simulink model "ModelTestVersion"  (Simulink 9.2)
settings: Solver=FixedStepAuto  StartTime=0.0  StopTime=30  FixedStep=0.01  RelTol=1e-3
values from neighbouring files (symbols this model uses):
  I = 1    [Initialization.m]
  Ke = 6.67*10e-4    (= 0.00667)    [Initialization.m]
  Kec = 8.33*10e-5    (= 0.000833)    [Initialization.m]
  Ki = 0.01    [Initialization.m]
  Kp = 0.015    [Initialization.m]
  P = 5    [Initialization.m]
libraries: simulink x2, fuzblock x1
settings Model: Creator=zelex  LastModifiedBy=zelex
settings DataIOCC: LimitDataPoints=off  SaveFormat=Dataset  SignalLoggingSaveFormat=Dataset
settings OptimizationCC: LifeSpan=auto
settings DebuggingCC: UnderspecifiedInitializationDetection=Simplified  MergeDetectMultiDrivingBlocksExec=error  FcnCallInpInsideContextMsg=error  StateNameClashWarn=none  SFUnexpectedBacktrackingDiag=error  SFNoUnconditionalDefaultTransitionDiag=error
settings HardwareCC: ProdBitPerPointer=64  ProdBitPerSizeT=64  ProdBitPerPtrDiffT=64  ProdLargestAtomicFloat=Float  ProdIntDivRoundTo=Zero  ProdEndianess=LittleEndian  ProdWordSize=64  ProdHWDeviceType=Intel->x86-64 (Windows64)
settings ModelReferenceCC: PropagateSignalLabelsOutOfModel=on
settings SFSimCC: SimUseLocalCustomCode=on
settings RTWCC: RTWUseLocalCustomCode=on
settings GRTTargetCC: GeneratePreprocessorConditionals=Use local settings  CombineOutputUpdateFcns=on  GRTInterface=off

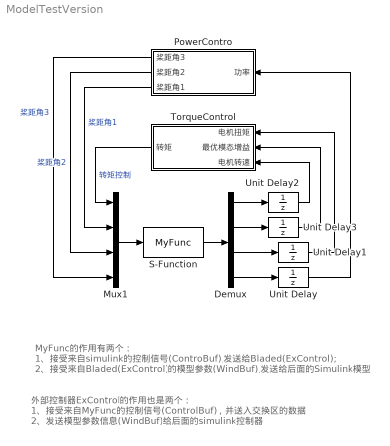
== system ModelTestVersion ==
  note: 外部控制器ExControl的作用也是两个：
      | 1、接受来自MyFunc的控制信号(ControlBuf)，并送入交换区的数据
      | 2、发送模型参数信息(WindBuf)给后面的simulink控制器
  note: MyFunc的作用有两个：
      | 1、接受来自simulink的控制信号(ControBuf),发送给Bladed(ExControl);
      | 2、接受来自Bladed(ExControl)的模型参数(WindBuf),发送给后面的Simulink模型
  Demux : Demux
  Mux1 : Mux
  PowerContro : Subsystem
  S-Function : S-Function  FunctionName=MyFunc  SFunctionDeploymentMode=off  EnableBusSupport=off
  TorqueControl : Subsystem
  Unit Delay : UnitDelay  SampleTime=0.01
  Unit Delay1 : UnitDelay  SampleTime=0.01
  Unit Delay2 : UnitDelay  SampleTime=0.01
  Unit Delay3 : UnitDelay  InitialCondition=22.82  SampleTime=0.01
  wires:
  Mux1/1 -> S-Function/1
  TorqueControl/1(转矩) -> Mux1/1  "转矩控制"
  PowerContro/3(桨距角1) -> Mux1/2  "桨距角1"
  PowerContro/2(桨距角2) -> Mux1/3  "桨距角2"
  PowerContro/1(桨距角3) -> Mux1/4  "桨距角3"
  S-Function/1 -> Demux/1
  Demux/1 -> Unit Delay2/1
  Demux/2 -> Unit Delay3/1
  Demux/3 -> Unit Delay1/1
  Demux/4 -> Unit Delay/1
  Unit Delay2/1 -> TorqueControl/3(电机转速)
  Unit Delay3/1 -> TorqueControl/2(最优模态增益)
  Unit Delay1/1 -> TorqueControl/1(电机扭矩)
  Unit Delay/1 -> PowerContro/1(功率)

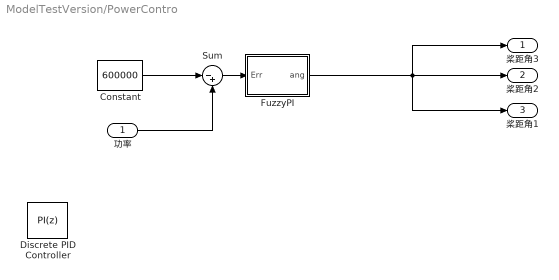
== system ModelTestVersion/PowerContro ==
  功率 : Inport
  Constant : Constant  Value=600000
  Discrete PID Controller : simulink/Continuous/PID Controller  Controller=PI  Form=Ideal  TimeDomain=Discrete-time  SampleTime=-1  IntegratorMethod=Forward Euler  FilterMethod=Forward Euler  ControllerParametersSource=internal  P=0.5  I=10  D=0  UseFilter=on  N=100  TunerSelectOption=Transfer Function Based (PID Tuner App)  InitialConditionSource=internal  InitialConditionForIntegrator=0  InitialConditionForFilter=0  DifferentiatorICPrevScaledInput=0  ExternalReset=none  TrackingMode=off  Kt=1  LimitOutput=off  UpperSaturationLimit=inf  LowerSaturationLimit=-inf  LinearizeAsGain=off  AntiWindupMode=none  Kb=1  POutMin=[]  POutMax=[]  IOutMin=[]  IOutMax=[]  DOutMin=[]  DOutMax=[]  NOutMin=[]  NOutMax=[]  SumOutMin=[]  SumOutMax=[]  SaturationOutMin=[]  SaturationOutMax=[]  PParamMin=[]  PParamMax=[]  IParamMin=[]  IParamMax=[]  DParamMin=[]  DParamMax=[]  NParamMin=[]  NParamMax=[]  KbParamMin=[]  KbParamMax=[]  KtParamMin=[]  KtParamMax=[]  KbOutMin=[]  KbOutMax=[]  KtOutMin=[]  KtOutMax=[]  IntegratorOutMin=[]  IntegratorOutMax=[]  FilterOutMin=[]  FilterOutMax=[]  SumI1OutMin=[]  SumI1OutMax=[]  SumI2OutMin=[]  SumI2OutMax=[]  SumI3OutMin=[]  SumI3OutMax=[]  SumI4OutMin=[]  SumI4OutMax=[]  SumDOutMin=[]  SumDOutMax=[]  DifferentiatorOutMin=[]  DifferentiatorOutMax=[]  FilterDiffOutCoefMin=[]  FilterDiffOutCoefMax=[]  ReciprocalOutMin=[]  ReciprocalOutMax=[]  SumDenOutMin=[]  SumDenOutMax=[]  SumNumOutMin=[]  SumNumOutMax=[]  DivideOutMin=[]  DivideOutMax=[]  IntegratorContinuousStateAttributes=''  IntegratorStateMustResolveToSignalObject=off  IntegratorRTWStateStorageClass=Auto  FilterContinuousStateAttributes=''  FilterStateMustResolveToSignalObject=off  FilterRTWStateStorageClass=Auto  ParallelPVariant=Passthrough  IdealPVariant=InternalParameters  IVariant=InternalParameters  DVariant=Disabled  IntegratorVariant=Discrete  SatVariant=Disabled  AWVariant=Passthrough  PCopyVariant=Disabled  TRVariant=Disabled  FdbkBlocksVariant=Forward  IdealPFdbkVariant=Disabled  SatFdbkVariant=Disabled  DerivativeFilterVariant=Disabled  NVariant=Disabled  NCopyVariant=Disabled_SignalSpec  FilterICVariant=Disabled  IntegratorICVariant=InternalICs  ExternalResetVariant=Disabled  TRSumVariant=Passthrough  SumFdbkVariant=Disabled  SumVariant=Sum_PI
  FuzzyPI : Subsystem
  Sum : Sum  Inputs=|-+
  桨距角3 : Outport
  桨距角2 : Outport  Port=2
  桨距角1 : Outport  Port=3
  wires:
  功率/1 -> Sum/2
  Constant/1 -> Sum/1
  FuzzyPI/1(ang) -> 桨距角1/1, 桨距角2/1, 桨距角3/1
  Sum/1 -> FuzzyPI/1(Err)

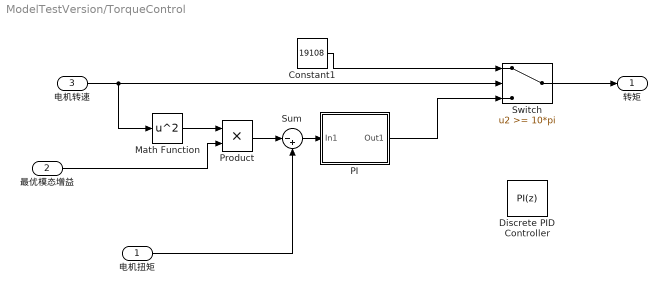
== system ModelTestVersion/TorqueControl ==
  电机扭矩 : Inport
  最优模态增益 : Inport  Port=2
  电机转速 : Inport  Port=3
  Constant1 : Constant  Value=19108
  Discrete PID Controller : simulink/Continuous/PID Controller  Controller=PI  Form=Ideal  TimeDomain=Discrete-time  SampleTime=-1  IntegratorMethod=Forward Euler  FilterMethod=Forward Euler  ControllerParametersSource=internal  P=100  I=2  D=0  UseFilter=on  N=100  TunerSelectOption=Transfer Function Based (PID Tuner App)  InitialConditionSource=internal  InitialConditionForIntegrator=0  InitialConditionForFilter=0  DifferentiatorICPrevScaledInput=0  ExternalReset=none  TrackingMode=off  Kt=1  LimitOutput=off  UpperSaturationLimit=inf  LowerSaturationLimit=-inf  LinearizeAsGain=off  AntiWindupMode=none  Kb=1  POutMin=[]  POutMax=[]  IOutMin=[]  IOutMax=[]  DOutMin=[]  DOutMax=[]  NOutMin=[]  NOutMax=[]  SumOutMin=[]  SumOutMax=[]  SaturationOutMin=[]  SaturationOutMax=[]  PParamMin=[]  PParamMax=[]  IParamMin=[]  IParamMax=[]  DParamMin=[]  DParamMax=[]  NParamMin=[]  NParamMax=[]  KbParamMin=[]  KbParamMax=[]  KtParamMin=[]  KtParamMax=[]  KbOutMin=[]  KbOutMax=[]  KtOutMin=[]  KtOutMax=[]  IntegratorOutMin=[]  IntegratorOutMax=[]  FilterOutMin=[]  FilterOutMax=[]  SumI1OutMin=[]  SumI1OutMax=[]  SumI2OutMin=[]  SumI2OutMax=[]  SumI3OutMin=[]  SumI3OutMax=[]  SumI4OutMin=[]  SumI4OutMax=[]  SumDOutMin=[]  SumDOutMax=[]  DifferentiatorOutMin=[]  DifferentiatorOutMax=[]  FilterDiffOutCoefMin=[]  FilterDiffOutCoefMax=[]  ReciprocalOutMin=[]  ReciprocalOutMax=[]  SumDenOutMin=[]  SumDenOutMax=[]  SumNumOutMin=[]  SumNumOutMax=[]  DivideOutMin=[]  DivideOutMax=[]  IntegratorContinuousStateAttributes=''  IntegratorStateMustResolveToSignalObject=off  IntegratorRTWStateStorageClass=Auto  FilterContinuousStateAttributes=''  FilterStateMustResolveToSignalObject=off  FilterRTWStateStorageClass=Auto  ParallelPVariant=Passthrough  IdealPVariant=InternalParameters  IVariant=InternalParameters  DVariant=Disabled  IntegratorVariant=Discrete  SatVariant=Disabled  AWVariant=Passthrough  PCopyVariant=Disabled  TRVariant=Disabled  FdbkBlocksVariant=Forward  IdealPFdbkVariant=Disabled  SatFdbkVariant=Disabled  DerivativeFilterVariant=Disabled  NVariant=Disabled  NCopyVariant=Disabled_SignalSpec  FilterICVariant=Disabled  IntegratorICVariant=InternalICs  ExternalResetVariant=Disabled  TRSumVariant=Passthrough  SumFdbkVariant=Disabled  SumVariant=Sum_PI
  Math Function : Math  Operator=square  SaturateOnIntegerOverflow=on
  PI : Subsystem
  Product : Product
  Sum : Sum  Inputs=|-+
  Switch : Switch  Threshold=10*pi
  转矩 : Outport
  wires:
  Switch/1 -> 转矩/1
  电机转速/1 -> Math Function/1, Switch/2
  最优模态增益/1 -> Product/2
  电机扭矩/1 -> Sum/2
  Constant1/1 -> Switch/1
  Math Function/1 -> Product/1
  Product/1 -> Sum/1
  Sum/1 -> PI/1(In1)
  PI/1(Out1) -> Switch/3

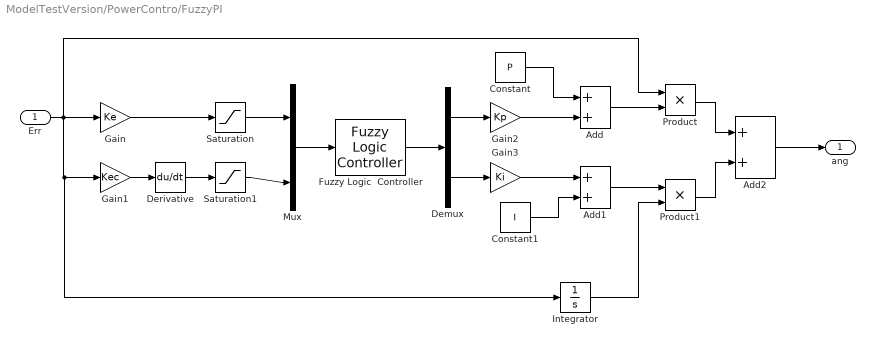
== system ModelTestVersion/PowerContro/FuzzyPI ==
  Err : Inport
  Add : Sum
  Add1 : Sum
  Add2 : Sum
  Constant : Constant  Value=P
  Constant1 : Constant  Value=I
  Demux : Demux  Outputs=2
  Derivative : Derivative
  Fuzzy Logic  Controller : fuzblock/Fuzzy Logic  Controller  FIS='fuzzpid.fis'  OutputSampleNumber=101  DataType=double  FuzzifiedInputs=off  RuleFiringStrengths=off  RuleOutputs=off  AggregatedOutputs=off  SimulateUsing=Interpreted execution  OutOfRangeInputValueMessage=warning  NoRuleFiredMessage=warning  EmptyOutputFuzzySetMessage=warning
  Gain : Gain  Gain=Ke
  Gain1 : Gain  Gain=Kec
  Gain2 : Gain  Gain=Kp
  Gain3 : Gain  Gain=Ki
  Integrator : Integrator
  Mux : Mux  Inputs=2
  Product : Product
  Product1 : Product
  Saturation : Saturate  UpperLimit=6  LowerLimit=-6
  Saturation1 : Saturate  UpperLimit=6  LowerLimit=-6
  ang : Outport
  wires:
  Err/1 -> Product/1, Integrator/1, Gain1/1, Gain/1
  Gain/1 -> Saturation/1
  Gain1/1 -> Derivative/1
  Derivative/1 -> Saturation1/1
  Saturation/1 -> Mux/1
  Saturation1/1 -> Mux/2
  Mux/1 -> Fuzzy Logic  Controller/1
  Fuzzy Logic  Controller/1 -> Demux/1
  Demux/1 -> Gain2/1
  Demux/2 -> Gain3/1
  Gain2/1 -> Add/2
  Constant/1 -> Add/1
  Gain3/1 -> Add1/1
  Constant1/1 -> Add1/2
  Integrator/1 -> Product1/2
  Add1/1 -> Product1/1
  Add/1 -> Product/2
  Add2/1 -> ang/1
  Product/1 -> Add2/1
  Product1/1 -> Add2/2

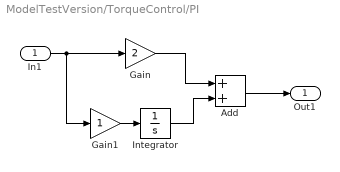
== system ModelTestVersion/TorqueControl/PI ==
  In1 : Inport
  Add : Sum
  Gain : Gain  Gain=2
  Gain1 : Gain
  Integrator : Integrator
  Out1 : Outport
  wires:
  In1/1 -> Gain1/1, Gain/1
  Gain1/1 -> Integrator/1
  Gain/1 -> Add/1
  Integrator/1 -> Add/2
  Add/1 -> Out1/1
